simulink model "ebike"  (Simulink 8.1)
settings: Solver=ode3  StartTime=0.0  StopTime=0.5  FixedStep=0.001  MaxStep=0.001  MinStep=0.001  RelTol=1e-3
values from neighbouring files (symbols this model uses):
  air_drag = 1.1    [RUN_SIM.M]
  area = 0.5    [RUN_SIM.M]
  roll_fric = 0.006    [RUN_SIM.M]
libraries: simulink x2
settings Model: Creator=stwei  LastModifiedBy=imrankp
settings DataIOCC: SignalLoggingSaveFormat=Dataset  SaveOutput=off  ReturnWorkspaceOutputs=on
settings GRTTargetCC: CodeReplacementLibrary=None  CPPClassGenCompliant=on

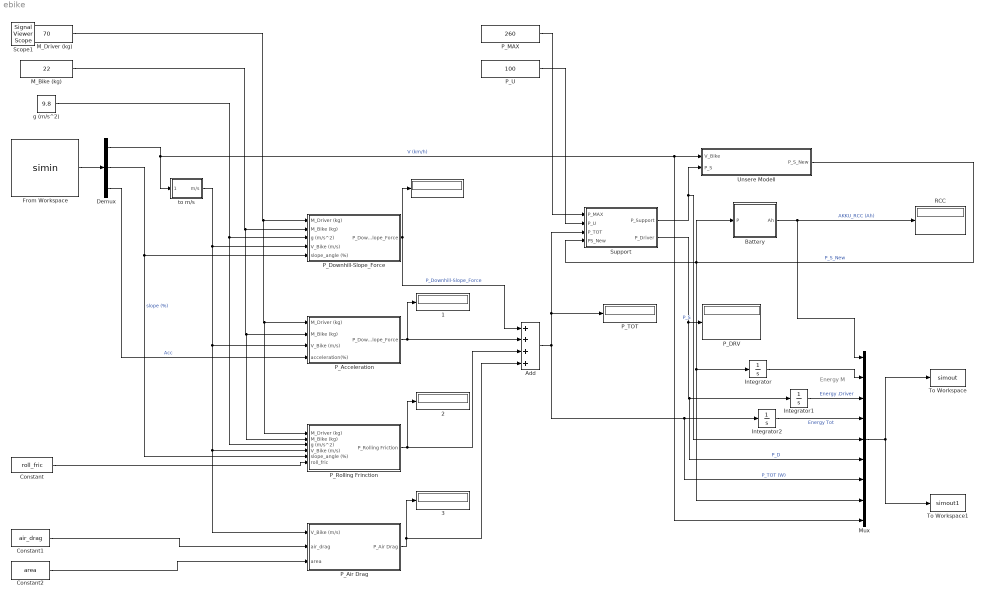
== system ebike ==
  note: Energy M
     {,1..3} (4 alike) : Display
  " P_DRV" : Display
  " P_TOT" : Display
  Add : Sum  Inputs=++++
  Battery : Subsystem
  Constant : Constant  Value=roll_fric
  Constant1 : Constant  Value=air_drag
  Constant2 : Constant  Value=area
  Demux : Demux  Outputs=3
  From Workspace : FromWorkspace  VariableName=simin  SampleTime=0  OutputAfterFinalValue=Setting to zero
  Integrator : Integrator
  Integrator1 : Integrator
  Integrator2 : Integrator
  M_Bike (kg) : Constant  Value=22
  M_Driver (kg) : Constant  Value=70
  Mux : Mux  Inputs=9
  P_Acceleration : Subsystem
  P_Air Drag : Subsystem
  P_Downhill-Slope_Force : Subsystem
  P_MAX : Constant  Value=260
  P_Rolling Frinction : Subsystem
  P_U : Constant  Value=100
  RCC : Display
  Support : Subsystem
  To Workspace : ToWorkspace  VariableName=simout  SampleTime=-1  SaveFormat=Structure With Time
  To Workspace1 : ToWorkspace  VariableName=simout1  SampleTime=-1  SaveFormat=Structure With Time
  Unsere Modell : Subsystem
  g (m/s^2) : Constant  Value=9.8
  to m/s : Subsystem
  Scope1 : SignalViewerScope  IOType=viewer  NumInputPorts=5  ZoomMode=xonly  RefreshTime=0.035000
      settings: ShowLegends=on  TimeRange=2  YMin=0~0~0~0~9  YMax=1000~1000~1000~60~13
  wires:
  M_Driver (kg)/1 -> P_Rolling Frinction/1(M_Driver (kg)), P_Acceleration/1(M_Driver (kg)), P_Downhill-Slope_Force/1(M_Driver (kg))
  M_Bike (kg)/1 -> P_Rolling Frinction/2(M_Bike (kg)), P_Acceleration/2(M_Bike (kg)), P_Downhill-Slope_Force/2(M_Bike (kg))
  g (m/s^2)/1 -> P_Rolling Frinction/3(g (m/s^2)), P_Downhill-Slope_Force/3(g (m/s^2))
  P_Downhill-Slope_Force/1(P_Downhill-Slope_Force) -> Add/1, "   "/1  "P_Downhill-Slope_Force"
  to m/s/1(m/s) -> P_Downhill-Slope_Force/4(V_Bike (m/s)), P_Acceleration/3(V_Bike (m/s)), P_Air Drag/1(V_Bike (m/s)), P_Rolling Frinction/4(V_Bike (m/s))
  P_MAX/1 -> Support/1(P_MAX)
  P_U/1 -> Support/2(P_U)
  Support/2(P_Driver) -> " P_DRV"/1, Mux/6, Integrator1/1  "P_D"
  Battery/1(Ah) -> RCC/1, Mux/1  "AKKU_RCC (Ah)"
  From Workspace/1 -> Demux/1
  Demux/1 -> to m/s/1(km/h), Mux/9, Unsere Modell/1(V_Bike)  "V (km/h)"
  Add/1 -> Integrator2/1, Mux/7, Support/3(P_TOT), " P_TOT"/1  "P_TOT (W)"
  Demux/2 -> P_Downhill-Slope_Force/5(slope_angle (%)), P_Rolling Frinction/5(slope_angle (%))  "slope (%)"
  Demux/3 -> P_Acceleration/4(acceleration(%))  "Acc"
  P_Acceleration/1(P_Downhill-Slope_Force) -> "   1"/1, Add/2
  P_Rolling Frinction/1(P_Rolling Friction) -> "   2"/1, Add/3
  P_Air Drag/1(P_Air Drag) -> "   3"/1, Add/4
  Mux/1 -> To Workspace/1, To Workspace1/1
  Constant/1 -> P_Rolling Frinction/6(roll_fric)
  Constant1/1 -> P_Air Drag/2(air_drag)
  Constant2/1 -> P_Air Drag/3(area)
  Integrator/1 -> Mux/2
  Integrator1/1 -> Mux/3  "Energy .Driver"
  Integrator2/1 -> Mux/4  "Energy Tot"
  Unsere Modell/1(P_S_New) -> Mux/8, Integrator/1, Battery/1(P), Support/4(PS_New)  "P_S_New"
  Support/1(P_Support) -> Mux/5, Unsere Modell/2(P_S)  "P_S"

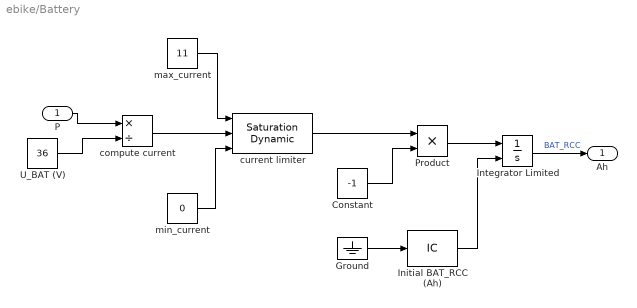
== system ebike/Battery ==
  P : Inport
  Constant : Constant  Value=-1
  Ground : Ground
  Initial BAT_RCC (Ah) : InitialCondition  Value=11
  Integrator Limited : Integrator  InitialConditionSource=external  LimitOutput=on  UpperSaturationLimit=13  LowerSaturationLimit=0
  Product : Product  RndMeth=Zero
  U_BAT (V) : Constant  Value=36
  compute current : Product  Inputs=*/
  current limiter : simulink/Discontinuities/Saturation Dynamic  OutMin=[]  OutMax=[]  OutDataTypeStr=Inherit: Same as second input  OutDataType=fixdt(1, 16)  OutScaling=2^-10  DoSatur=on
  max_current : Constant  Value=11
  min_current : Constant  Value=0
  Ah : Outport
  wires:
  Ground/1 -> Initial BAT_RCC (Ah)/1
  U_BAT (V)/1 -> compute current/2
  Initial BAT_RCC (Ah)/1 -> Integrator Limited/2
  Constant/1 -> Product/2
  Product/1 -> Integrator Limited/1
  P/1 -> compute current/1
  Integrator Limited/1 -> Ah/1  "BAT_RCC"
  current limiter/1 -> Product/1
  compute current/1 -> current limiter/2
  max_current/1 -> current limiter/1
  min_current/1 -> current limiter/3

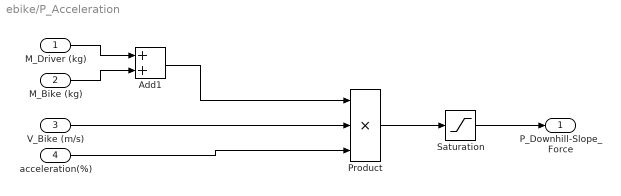
== system ebike/P_Acceleration ==
  M_Driver (kg) : Inport
  M_Bike (kg) : Inport  Port=2
  V_Bike (m/s) : Inport  Port=3
  acceleration(%) : Inport  Port=4
  Add1 : Sum
  Product : Product  Inputs=3  RndMeth=Zero
  Saturation : Saturate  UpperLimit=10000  LowerLimit=0
  P_Downhill-Slope_Force : Outport
  wires:
  Add1/1 -> Product/1
  M_Driver (kg)/1 -> Add1/1
  M_Bike (kg)/1 -> Add1/2
  V_Bike (m/s)/1 -> Product/2
  acceleration(%)/1 -> Product/3
  Product/1 -> Saturation/1
  Saturation/1 -> P_Downhill-Slope_Force/1

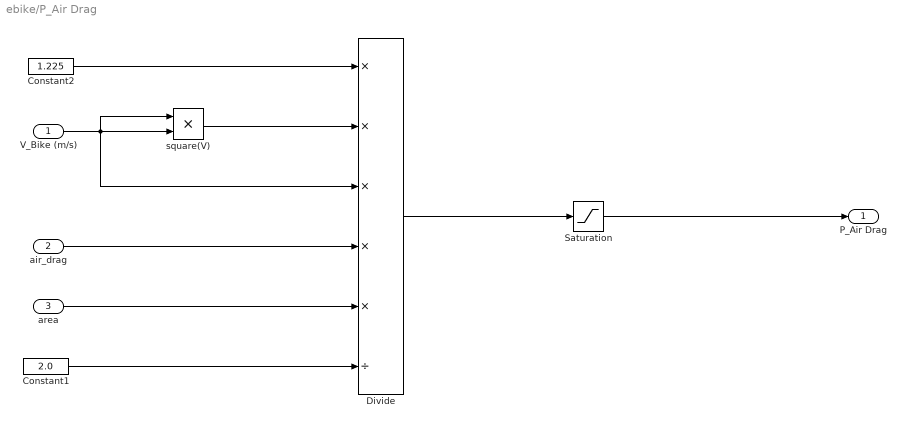
== system ebike/P_Air Drag ==
  V_Bike (m/s) : Inport
  air_drag : Inport  Port=2
  area : Inport  Port=3
  Constant1 : Constant  Value=2.0
  Constant2 : Constant  Value=1.225
  Divide : Product  Inputs=*****/
  Saturation : Saturate  UpperLimit=10000  LowerLimit=0
  square(V) : Product
  P_Air Drag : Outport
  wires:
  Saturation/1 -> P_Air Drag/1
  V_Bike (m/s)/1 -> Divide/3, square(V)/1, square(V)/2
  Constant2/1 -> Divide/1
  air_drag/1 -> Divide/4
  area/1 -> Divide/5
  square(V)/1 -> Divide/2
  Divide/1 -> Saturation/1
  Constant1/1 -> Divide/6

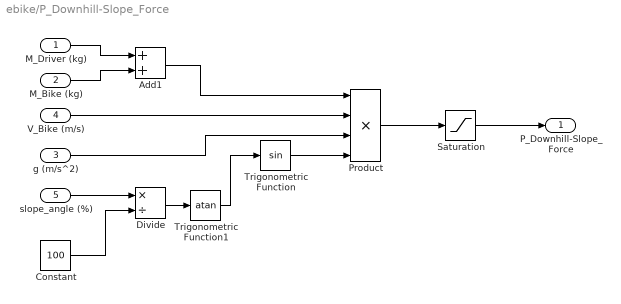
== system ebike/P_Downhill-Slope_Force ==
  M_Driver (kg) : Inport
  M_Bike (kg) : Inport  Port=2
  g (m/s^2) : Inport  Port=3
  V_Bike (m/s) : Inport  Port=4
  slope_angle (%) : Inport  Port=5
  Add1 : Sum
  Constant : Constant  Value=100
  Divide : Product  Inputs=*/
  Product : Product  Inputs=4  RndMeth=Zero
  Saturation : Saturate  UpperLimit=10000  LowerLimit=0
  Trigonometric Function : Trigonometry
  Trigonometric Function1 : Trigonometry  Operator=atan
  P_Downhill-Slope_Force : Outport
  wires:
  Add1/1 -> Product/1
  M_Driver (kg)/1 -> Add1/1
  M_Bike (kg)/1 -> Add1/2
  V_Bike (m/s)/1 -> Product/2
  g (m/s^2)/1 -> Product/3
  Trigonometric Function/1 -> Product/4
  Trigonometric Function1/1 -> Trigonometric Function/1
  slope_angle (%)/1 -> Divide/1
  Divide/1 -> Trigonometric Function1/1
  Constant/1 -> Divide/2
  Product/1 -> Saturation/1
  Saturation/1 -> P_Downhill-Slope_Force/1

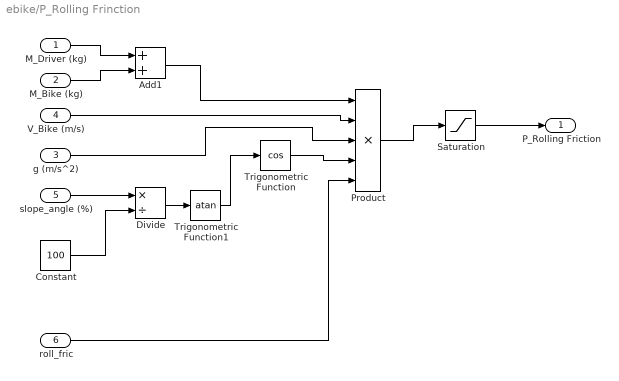
== system ebike/P_Rolling Frinction ==
  M_Driver (kg) : Inport
  M_Bike (kg) : Inport  Port=2
  g (m/s^2) : Inport  Port=3
  V_Bike (m/s) : Inport  Port=4
  slope_angle (%) : Inport  Port=5
  roll_fric : Inport  Port=6
  Add1 : Sum
  Constant : Constant  Value=100
  Divide : Product  Inputs=*/
  Product : Product  Inputs=5  RndMeth=Zero
  Saturation : Saturate  UpperLimit=10000  LowerLimit=0
  Trigonometric Function : Trigonometry  Operator=cos
  Trigonometric Function1 : Trigonometry  Operator=atan
  P_Rolling Friction : Outport
  wires:
  Add1/1 -> Product/1
  M_Driver (kg)/1 -> Add1/1
  M_Bike (kg)/1 -> Add1/2
  V_Bike (m/s)/1 -> Product/2
  g (m/s^2)/1 -> Product/3
  Trigonometric Function/1 -> Product/4
  Trigonometric Function1/1 -> Trigonometric Function/1
  slope_angle (%)/1 -> Divide/1
  Divide/1 -> Trigonometric Function1/1
  Constant/1 -> Divide/2
  Product/1 -> Saturation/1
  Saturation/1 -> P_Rolling Friction/1
  roll_fric/1 -> Product/5

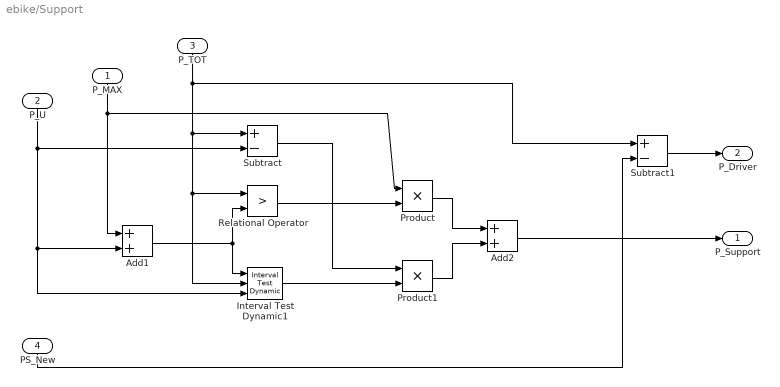
== system ebike/Support ==
  P_MAX : Inport
  P_U : Inport  Port=2
  P_TOT : Inport  Port=3
  PS_New : Inport  Port=4
  Add1 : Sum
  Add2 : Sum
  Interval Test Dynamic1 : simulink/Logic and Bit Operations/Interval Test Dynamic  IntervalClosedRight=on  IntervalClosedLeft=on  OutDataTypeStr=uint8
  Product : Product  RndMeth=Zero
  Product1 : Product  RndMeth=Zero
  Relational Operator : RelationalOperator  Operator=>  OutDataTypeStr=boolean
  Subtract : Sum  Inputs=+-
  Subtract1 : Sum  Inputs=+-
  P_Support : Outport
  P_Driver : Outport  Port=2
  wires:
  Add1/1 -> Interval Test Dynamic1/1, Relational Operator/2
  P_TOT/1 -> Subtract1/1, Subtract/1, Interval Test Dynamic1/2, Relational Operator/1
  P_U/1 -> Subtract/2, Interval Test Dynamic1/3, Add1/2
  P_MAX/1 -> Product/1, Add1/1
  Relational Operator/1 -> Product/2
  Subtract/1 -> Product1/1
  Interval Test Dynamic1/1 -> Product1/2
  Product/1 -> Add2/1
  Product1/1 -> Add2/2
  Add2/1 -> P_Support/1
  Subtract1/1 -> P_Driver/1
  PS_New/1 -> Subtract1/2

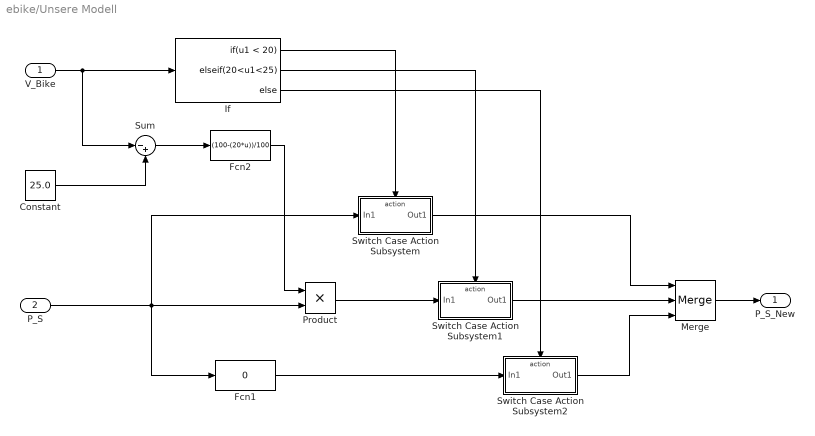
== system ebike/Unsere Modell ==
  V_Bike : Inport
  P_S : Inport  Port=2
  Constant : Constant  Value=25.0
  Fcn1 : Fcn  Expr=0
  Fcn2 : Fcn  Expr=(100-(20*u))/100
  If : If  IfExpression=u1 < 20  ElseIfExpressions=20<u1<25
  Merge : Merge  Inputs=3  InitialOutput=0  AllowUnequalInputPortWidths=on
  Product : Product
  Sum : Sum  Inputs=|-+
  Switch Case Action Subsystem : Subsystem  TreatAsAtomicUnit=on
  Switch Case Action Subsystem1 : Subsystem  TreatAsAtomicUnit=on
  Switch Case Action Subsystem2 : Subsystem  TreatAsAtomicUnit=on
  P_S_New : Outport
  wires:
  P_S/1 -> Fcn1/1, Switch Case Action Subsystem/1(In1), Product/2
  V_Bike/1 -> Sum/1, If/1
  Constant/1 -> Sum/2
  Sum/1 -> Fcn2/1
  If/1 -> Switch Case Action Subsystem/Action
  If/2 -> Switch Case Action Subsystem1/Action
  If/3 -> Switch Case Action Subsystem2/Action
  Switch Case Action Subsystem/1(Out1) -> Merge/1
  Merge/1 -> P_S_New/1
  Fcn2/1 -> Product/1
  Product/1 -> Switch Case Action Subsystem1/1(In1)
  Switch Case Action Subsystem1/1(Out1) -> Merge/2
  Fcn1/1 -> Switch Case Action Subsystem2/1(In1)
  Switch Case Action Subsystem2/1(Out1) -> Merge/3

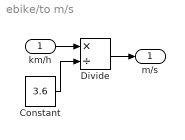
== system ebike/to m/s ==
  km/h : Inport
  Constant : Constant  Value=3.6
  Divide : Product  Inputs=*/
  m/s : Outport
  wires:
  Constant/1 -> Divide/2
  km/h/1 -> Divide/1
  Divide/1 -> m/s/1

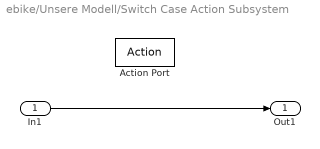
== system ebike/Unsere Modell/Switch Case Action Subsystem ==
  In1 : Inport
  Action Port : ActionPort  InitializeStates=reset  ActionType=then
  Out1 : Outport
  wires:
  In1/1 -> Out1/1

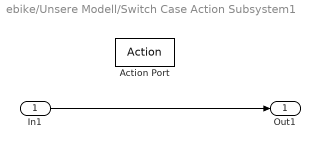
== system ebike/Unsere Modell/Switch Case Action Subsystem1 ==
  In1 : Inport
  Action Port : ActionPort  InitializeStates=reset  ActionType=elseif
  Out1 : Outport
  wires:
  In1/1 -> Out1/1

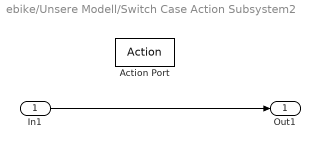
== system ebike/Unsere Modell/Switch Case Action Subsystem2 ==
  In1 : Inport
  Action Port : ActionPort  InitializeStates=reset  ActionType=else
  Out1 : Outport
  wires:
  In1/1 -> Out1/1
